simulink model "xblock_half_band_Model"  (Simulink 7.4)
settings: Solver=ode45  StartTime=0.0  StopTime=10.0  RelTol=1e-3
libraries: xbsIndex_r4 x629, casper_library_misc x12
(part 1 of 6)
settings Model: Creator=hong  LastModifiedBy=hong

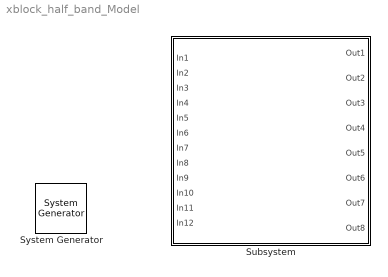
== system xblock_half_band_Model ==
  " System Generator" : xbsIndex_r4/ System Generator  Tag=genX  SystemSampleTime=-1  xilinxfamily=Virtex6  part=xc6vsx315t  speed=-3  package=ff1156  synthesis_tool=XST  clock_wrapper=Clock Enables  directory=./netlist  testbench=off  simulink_period=1  sysclk_period=10  dcm_input_clock_period=10  incr_netlist=off  trim_vbits=Everywhere in SubSystem  dbl_ovrd=According to Block Masks  core_generation=According to Block Masks  run_coregen=off  deprecated_control=off  eval_field=0  block_type=sysgen
      settings: block_version=11.4
  Subsystem : Subsystem

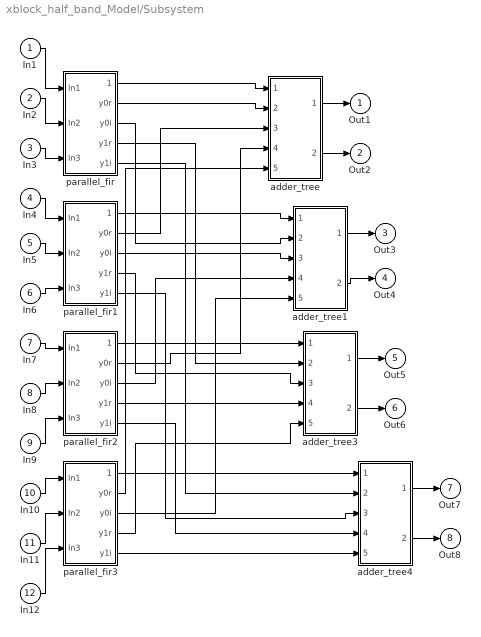
== system xblock_half_band_Model/Subsystem ==
  In1 : Inport
  In2 : Inport  Port=2
  In3 : Inport  Port=3
  In4 : Inport  Port=4
  In5 : Inport  Port=5
  In6 : Inport  Port=6
  In7 : Inport  Port=7
  In8 : Inport  Port=8
  In9 : Inport  Port=9
  In10 : Inport  Port=10
  In11 : Inport  Port=11
  In12 : Inport  Port=12
  adder_tree : Subsystem
  adder_tree1 : Subsystem
  adder_tree3 : Subsystem
  adder_tree4 : Subsystem
  parallel_fir : Subsystem
  parallel_fir1 : Subsystem
  parallel_fir2 : Subsystem
  parallel_fir3 : Subsystem
  Out1 : Outport
  Out2 : Outport  Port=2
  Out3 : Outport  Port=3
  Out4 : Outport  Port=4
  Out5 : Outport  Port=5
  Out6 : Outport  Port=6
  Out7 : Outport  Port=7
  Out8 : Outport  Port=8
  wires:
  parallel_fir3/4(y1r) -> adder_tree3/5(din_4)
  parallel_fir3/2(y0r) -> adder_tree/5(din_4)
  In12/1 -> parallel_fir3/3(In3)
  In10/1 -> parallel_fir3/1(In1)
  parallel_fir2/5(y1i) -> adder_tree4/4(din_3)
  parallel_fir2/3(y0i) -> adder_tree1/4(din_3)
  parallel_fir2/1(sync_out) -> adder_tree3/1(sync)
  In8/1 -> parallel_fir2/2(In2)
  parallel_fir1/4(y1r) -> adder_tree3/3(din_2)
  parallel_fir1/2(y0r) -> adder_tree/3(din_2)
  In6/1 -> parallel_fir1/3(In3)
  In4/1 -> parallel_fir1/1(In1)
  parallel_fir/5(y1i) -> adder_tree4/2(din_1)
  parallel_fir/3(y0i) -> adder_tree1/2(din_1)
  parallel_fir/1(sync_out) -> adder_tree/1(sync)
  In2/1 -> parallel_fir/2(In2)
  adder_tree4/1(sync_out) -> Out7/1
  adder_tree3/2(dout) -> Out6/1
  adder_tree1/1(sync_out) -> Out3/1
  adder_tree/2(dout) -> Out2/1
  adder_tree/1(sync_out) -> Out1/1
  adder_tree1/2(dout) -> Out4/1
  adder_tree3/1(sync_out) -> Out5/1
  adder_tree4/2(dout) -> Out8/1
  In1/1 -> parallel_fir/1(In1)
  In3/1 -> parallel_fir/3(In3)
  parallel_fir/2(y0r) -> adder_tree/2(din_1)
  parallel_fir/4(y1r) -> adder_tree3/2(din_1)
  In5/1 -> parallel_fir1/2(In2)
  parallel_fir1/1(sync_out) -> adder_tree1/1(sync)
  parallel_fir1/3(y0i) -> adder_tree1/3(din_2)
  parallel_fir1/5(y1i) -> adder_tree4/3(din_2)
  In7/1 -> parallel_fir2/1(In1)
  In9/1 -> parallel_fir2/3(In3)
  parallel_fir2/2(y0r) -> adder_tree/4(din_3)
  parallel_fir2/4(y1r) -> adder_tree3/4(din_3)
  In11/1 -> parallel_fir3/2(In2)
  parallel_fir3/1(sync_out) -> adder_tree4/1(sync)
  parallel_fir3/3(y0i) -> adder_tree1/5(din_4)
  parallel_fir3/5(y1i) -> adder_tree4/5(din_4)

== system xblock_half_band_Model/Subsystem/adder_tree ==
  sync : Inport
  din_1 : Inport  Port=2
  din_2 : Inport  Port=3
  din_3 : Inport  Port=4
  din_4 : Inport  Port=5
  adder_0 : xbsIndex_r4/AddSub  mode=Addition  use_carryin=off  use_carryout=off  en=off  latency=1  precision=Full  arith_type=Unsigned  n_bits=16  bin_pt=14  quantization=Truncate  overflow=Saturate  dbl_ovrd=off  use_behavioral_HDL=off  hw_selection=Fabric  pipelined=off  block_type=addsub
  adder_1 : xbsIndex_r4/AddSub  mode=Addition  use_carryin=off  use_carryout=off  en=off  latency=1  precision=Full  arith_type=Unsigned  n_bits=16  bin_pt=14  quantization=Truncate  overflow=Saturate  dbl_ovrd=off  use_behavioral_HDL=off  hw_selection=Fabric  pipelined=off  block_type=addsub
  adder_2 : xbsIndex_r4/AddSub  mode=Addition  use_carryin=off  use_carryout=off  en=off  latency=1  precision=Full  arith_type=Unsigned  n_bits=16  bin_pt=14  quantization=Truncate  overflow=Saturate  dbl_ovrd=off  use_behavioral_HDL=off  hw_selection=Fabric  pipelined=off  block_type=addsub
  sync_delay : xbsIndex_r4/Delay  en=off  latency=2  dbl_ovrd=off  reg_retiming=off  block_type=delay
      settings: block_version=11.4
  zero_in : xbsIndex_r4/Constant  arith_type=Unsigned  const=0  n_bits=18  bin_pt=17  explicit_period=off  period=1  equ=P=C  opselect=C  inp2=PCIN>>17  opr=+  inp1=P  carry=CIN  dbl_ovrd=off  block_type=constant
      settings: block_version=11.4
  sync_out : Outport
  dout : Outport  Port=2
  wires:
  adder_0/1 -> adder_2/2
  din_4/1 -> adder_1/1
  din_1/1 -> adder_0/2
  sync/1 -> sync_delay/1
  sync_delay/1 -> sync_out/1
  din_2/1 -> adder_0/1
  din_3/1 -> adder_1/2
  adder_1/1 -> adder_2/1
  adder_2/1 -> dout/1

== system xblock_half_band_Model/Subsystem/adder_tree1 ==
  sync : Inport
  din_1 : Inport  Port=2
  din_2 : Inport  Port=3
  din_3 : Inport  Port=4
  din_4 : Inport  Port=5
  adder_0 : xbsIndex_r4/AddSub  mode=Addition  use_carryin=off  use_carryout=off  en=off  latency=1  precision=Full  arith_type=Unsigned  n_bits=16  bin_pt=14  quantization=Truncate  overflow=Saturate  dbl_ovrd=off  use_behavioral_HDL=off  hw_selection=Fabric  pipelined=off  block_type=addsub
  adder_1 : xbsIndex_r4/AddSub  mode=Addition  use_carryin=off  use_carryout=off  en=off  latency=1  precision=Full  arith_type=Unsigned  n_bits=16  bin_pt=14  quantization=Truncate  overflow=Saturate  dbl_ovrd=off  use_behavioral_HDL=off  hw_selection=Fabric  pipelined=off  block_type=addsub
  adder_2 : xbsIndex_r4/AddSub  mode=Addition  use_carryin=off  use_carryout=off  en=off  latency=1  precision=Full  arith_type=Unsigned  n_bits=16  bin_pt=14  quantization=Truncate  overflow=Saturate  dbl_ovrd=off  use_behavioral_HDL=off  hw_selection=Fabric  pipelined=off  block_type=addsub
  sync_delay : xbsIndex_r4/Delay  en=off  latency=2  dbl_ovrd=off  reg_retiming=off  block_type=delay
      settings: block_version=11.4
  zero_in : xbsIndex_r4/Constant  arith_type=Unsigned  const=0  n_bits=18  bin_pt=17  explicit_period=off  period=1  equ=P=C  opselect=C  inp2=PCIN>>17  opr=+  inp1=P  carry=CIN  dbl_ovrd=off  block_type=constant
      settings: block_version=11.4
  sync_out : Outport
  dout : Outport  Port=2
  wires:
  adder_0/1 -> adder_2/2
  din_4/1 -> adder_1/1
  din_1/1 -> adder_0/2
  sync/1 -> sync_delay/1
  sync_delay/1 -> sync_out/1
  din_2/1 -> adder_0/1
  din_3/1 -> adder_1/2
  adder_1/1 -> adder_2/1
  adder_2/1 -> dout/1

== system xblock_half_band_Model/Subsystem/adder_tree3 ==
  sync : Inport
  din_1 : Inport  Port=2
  din_2 : Inport  Port=3
  din_3 : Inport  Port=4
  din_4 : Inport  Port=5
  adder_0 : xbsIndex_r4/AddSub  mode=Addition  use_carryin=off  use_carryout=off  en=off  latency=1  precision=Full  arith_type=Unsigned  n_bits=16  bin_pt=14  quantization=Truncate  overflow=Saturate  dbl_ovrd=off  use_behavioral_HDL=off  hw_selection=Fabric  pipelined=off  block_type=addsub
  adder_1 : xbsIndex_r4/AddSub  mode=Addition  use_carryin=off  use_carryout=off  en=off  latency=1  precision=Full  arith_type=Unsigned  n_bits=16  bin_pt=14  quantization=Truncate  overflow=Saturate  dbl_ovrd=off  use_behavioral_HDL=off  hw_selection=Fabric  pipelined=off  block_type=addsub
  adder_2 : xbsIndex_r4/AddSub  mode=Addition  use_carryin=off  use_carryout=off  en=off  latency=1  precision=Full  arith_type=Unsigned  n_bits=16  bin_pt=14  quantization=Truncate  overflow=Saturate  dbl_ovrd=off  use_behavioral_HDL=off  hw_selection=Fabric  pipelined=off  block_type=addsub
  sync_delay : xbsIndex_r4/Delay  en=off  latency=2  dbl_ovrd=off  reg_retiming=off  block_type=delay
      settings: block_version=11.4
  zero_in : xbsIndex_r4/Constant  arith_type=Unsigned  const=0  n_bits=18  bin_pt=17  explicit_period=off  period=1  equ=P=C  opselect=C  inp2=PCIN>>17  opr=+  inp1=P  carry=CIN  dbl_ovrd=off  block_type=constant
      settings: block_version=11.4
  sync_out : Outport
  dout : Outport  Port=2
  wires:
  adder_0/1 -> adder_2/2
  din_4/1 -> adder_1/1
  din_1/1 -> adder_0/2
  sync/1 -> sync_delay/1
  sync_delay/1 -> sync_out/1
  din_2/1 -> adder_0/1
  din_3/1 -> adder_1/2
  adder_1/1 -> adder_2/1
  adder_2/1 -> dout/1

== system xblock_half_band_Model/Subsystem/adder_tree4 ==
  sync : Inport
  din_1 : Inport  Port=2
  din_2 : Inport  Port=3
  din_3 : Inport  Port=4
  din_4 : Inport  Port=5
  adder_0 : xbsIndex_r4/AddSub  mode=Addition  use_carryin=off  use_carryout=off  en=off  latency=1  precision=Full  arith_type=Unsigned  n_bits=16  bin_pt=14  quantization=Truncate  overflow=Saturate  dbl_ovrd=off  use_behavioral_HDL=off  hw_selection=Fabric  pipelined=off  block_type=addsub
  adder_1 : xbsIndex_r4/AddSub  mode=Addition  use_carryin=off  use_carryout=off  en=off  latency=1  precision=Full  arith_type=Unsigned  n_bits=16  bin_pt=14  quantization=Truncate  overflow=Saturate  dbl_ovrd=off  use_behavioral_HDL=off  hw_selection=Fabric  pipelined=off  block_type=addsub
  adder_2 : xbsIndex_r4/AddSub  mode=Addition  use_carryin=off  use_carryout=off  en=off  latency=1  precision=Full  arith_type=Unsigned  n_bits=16  bin_pt=14  quantization=Truncate  overflow=Saturate  dbl_ovrd=off  use_behavioral_HDL=off  hw_selection=Fabric  pipelined=off  block_type=addsub
  sync_delay : xbsIndex_r4/Delay  en=off  latency=2  dbl_ovrd=off  reg_retiming=off  block_type=delay
      settings: block_version=11.4
  zero_in : xbsIndex_r4/Constant  arith_type=Unsigned  const=0  n_bits=18  bin_pt=17  explicit_period=off  period=1  equ=P=C  opselect=C  inp2=PCIN>>17  opr=+  inp1=P  carry=CIN  dbl_ovrd=off  block_type=constant
      settings: block_version=11.4
  sync_out : Outport
  dout : Outport  Port=2
  wires:
  adder_0/1 -> adder_2/2
  din_4/1 -> adder_1/1
  din_1/1 -> adder_0/2
  sync/1 -> sync_delay/1
  sync_delay/1 -> sync_out/1
  din_2/1 -> adder_0/1
  din_3/1 -> adder_1/2
  adder_1/1 -> adder_2/1
  adder_2/1 -> dout/1

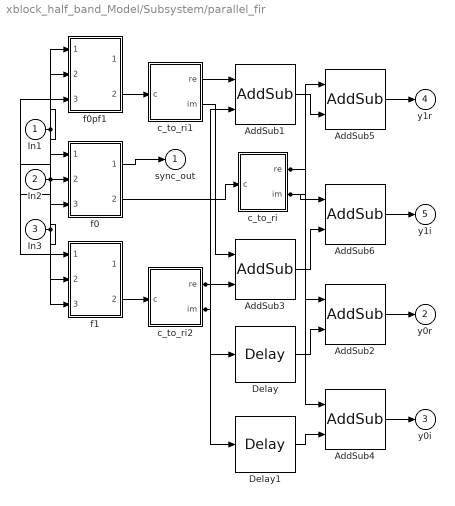
== system xblock_half_band_Model/Subsystem/parallel_fir ==
  In1 : Inport
  In2 : Inport  Port=2
  In3 : Inport  Port=3
  AddSub{1,3,5..6} (4 alike) : xbsIndex_r4/AddSub  mode=Subtraction  use_carryin=off  use_carryout=off  en=off  latency=0  precision=Full  arith_type=Unsigned  n_bits=16  bin_pt=14  quantization=Truncate  overflow=Wrap  dbl_ovrd=off  use_behavioral_HDL=off  hw_selection=Fabric  pipelined=off  block_type=addsub
  AddSub2 : xbsIndex_r4/AddSub  mode=Addition  use_carryin=off  use_carryout=off  en=off  latency=0  precision=Full  arith_type=Unsigned  n_bits=16  bin_pt=14  quantization=Truncate  overflow=Wrap  dbl_ovrd=off  use_behavioral_HDL=off  hw_selection=Fabric  pipelined=off  block_type=addsub
  AddSub4 : xbsIndex_r4/AddSub  mode=Addition  use_carryin=off  use_carryout=off  en=off  latency=0  precision=Full  arith_type=Unsigned  n_bits=16  bin_pt=14  quantization=Truncate  overflow=Wrap  dbl_ovrd=off  use_behavioral_HDL=off  hw_selection=Fabric  pipelined=off  block_type=addsub
  Delay : xbsIndex_r4/Delay  en=off  latency=1  dbl_ovrd=off  reg_retiming=off  block_type=delay
      settings: block_version=11.4
  Delay1 : xbsIndex_r4/Delay  en=off  latency=1  dbl_ovrd=off  reg_retiming=off  block_type=delay
      settings: block_version=11.4
  c_to_ri : Subsystem
  c_to_ri1 : Subsystem
  c_to_ri2 : Subsystem
  f0 : Subsystem
  f0pf1 : Subsystem
  f1 : Subsystem
  sync_out : Outport
  y0r : Outport  Port=2
  y0i : Outport  Port=3
  y1r : Outport  Port=4
  y1i : Outport  Port=5
  wires:
  c_to_ri/1(re) -> AddSub5/1, AddSub2/1
  c_to_ri/2(im) -> AddSub4/1, AddSub6/1
  c_to_ri2/1(re) -> Delay/1, AddSub1/2
  c_to_ri2/2(im) -> AddSub3/2, Delay1/1
  In1/1 -> f1/1(sync_in), f0/1(sync_in), f0pf1/1(sync_in)
  In2/1 -> f0pf1/2(real1), f0/2(real1), f1/2(real1)
  In3/1 -> f1/3(imag1), f0/3(imag1), f0pf1/3(imag1)
  f0pf1/2(dout) -> c_to_ri1/1(c)
  f0/1(sync_out) -> sync_out/1
  c_to_ri1/2(im) -> AddSub3/1
  Delay1/1 -> AddSub4/2
  Delay/1 -> AddSub2/2
  AddSub6/1 -> y1i/1
  AddSub1/1 -> AddSub5/2
  AddSub4/1 -> y0i/1
  AddSub2/1 -> y0r/1
  AddSub5/1 -> y1r/1
  AddSub3/1 -> AddSub6/2
  c_to_ri1/1(re) -> AddSub1/1
  f0/2(dout) -> c_to_ri/1(c)
  f1/2(dout) -> c_to_ri2/1(c)

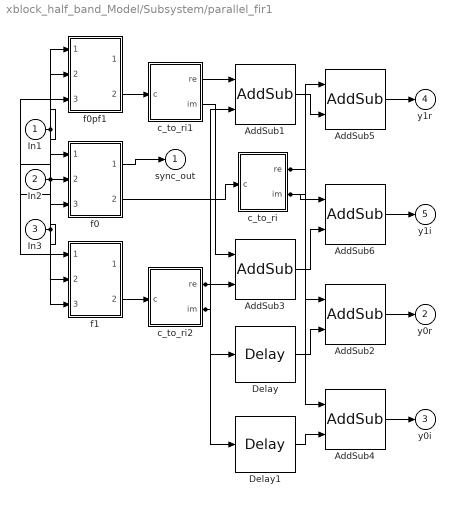
== system xblock_half_band_Model/Subsystem/parallel_fir1 ==
  In1 : Inport
  In2 : Inport  Port=2
  In3 : Inport  Port=3
  AddSub{1,3,5..6} (4 alike) : xbsIndex_r4/AddSub  mode=Subtraction  use_carryin=off  use_carryout=off  en=off  latency=0  precision=Full  arith_type=Unsigned  n_bits=16  bin_pt=14  quantization=Truncate  overflow=Wrap  dbl_ovrd=off  use_behavioral_HDL=off  hw_selection=Fabric  pipelined=off  block_type=addsub
  AddSub2 : xbsIndex_r4/AddSub  mode=Addition  use_carryin=off  use_carryout=off  en=off  latency=0  precision=Full  arith_type=Unsigned  n_bits=16  bin_pt=14  quantization=Truncate  overflow=Wrap  dbl_ovrd=off  use_behavioral_HDL=off  hw_selection=Fabric  pipelined=off  block_type=addsub
  AddSub4 : xbsIndex_r4/AddSub  mode=Addition  use_carryin=off  use_carryout=off  en=off  latency=0  precision=Full  arith_type=Unsigned  n_bits=16  bin_pt=14  quantization=Truncate  overflow=Wrap  dbl_ovrd=off  use_behavioral_HDL=off  hw_selection=Fabric  pipelined=off  block_type=addsub
  Delay : xbsIndex_r4/Delay  en=off  latency=1  dbl_ovrd=off  reg_retiming=off  block_type=delay
      settings: block_version=11.4
  Delay1 : xbsIndex_r4/Delay  en=off  latency=1  dbl_ovrd=off  reg_retiming=off  block_type=delay
      settings: block_version=11.4
  c_to_ri : Subsystem
  c_to_ri1 : Subsystem
  c_to_ri2 : Subsystem
  f0 : Subsystem
  f0pf1 : Subsystem
  f1 : Subsystem
  sync_out : Outport
  y0r : Outport  Port=2
  y0i : Outport  Port=3
  y1r : Outport  Port=4
  y1i : Outport  Port=5
  wires:
  c_to_ri/1(re) -> AddSub5/1, AddSub2/1
  c_to_ri/2(im) -> AddSub4/1, AddSub6/1
  c_to_ri2/1(re) -> Delay/1, AddSub1/2
  c_to_ri2/2(im) -> AddSub3/2, Delay1/1
  In1/1 -> f1/1(sync_in), f0/1(sync_in), f0pf1/1(sync_in)
  In2/1 -> f0pf1/2(real1), f0/2(real1), f1/2(real1)
  In3/1 -> f1/3(imag1), f0/3(imag1), f0pf1/3(imag1)
  f0pf1/2(dout) -> c_to_ri1/1(c)
  f0/1(sync_out) -> sync_out/1
  c_to_ri1/2(im) -> AddSub3/1
  Delay1/1 -> AddSub4/2
  Delay/1 -> AddSub2/2
  AddSub6/1 -> y1i/1
  AddSub1/1 -> AddSub5/2
  AddSub4/1 -> y0i/1
  AddSub2/1 -> y0r/1
  AddSub5/1 -> y1r/1
  AddSub3/1 -> AddSub6/2
  c_to_ri1/1(re) -> AddSub1/1
  f0/2(dout) -> c_to_ri/1(c)
  f1/2(dout) -> c_to_ri2/1(c)

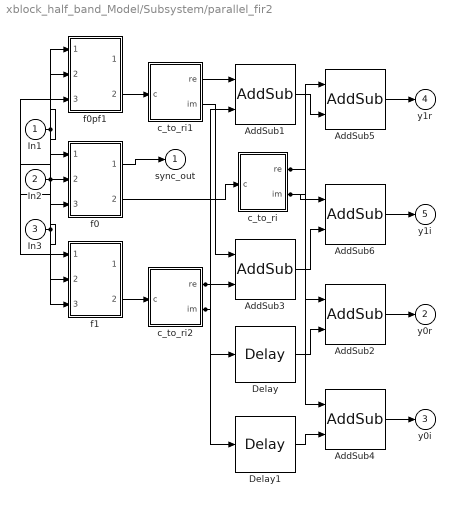
== system xblock_half_band_Model/Subsystem/parallel_fir2 ==
  In1 : Inport
  In2 : Inport  Port=2
  In3 : Inport  Port=3
  AddSub{1,3,5..6} (4 alike) : xbsIndex_r4/AddSub  mode=Subtraction  use_carryin=off  use_carryout=off  en=off  latency=0  precision=Full  arith_type=Unsigned  n_bits=16  bin_pt=14  quantization=Truncate  overflow=Wrap  dbl_ovrd=off  use_behavioral_HDL=off  hw_selection=Fabric  pipelined=off  block_type=addsub
  AddSub2 : xbsIndex_r4/AddSub  mode=Addition  use_carryin=off  use_carryout=off  en=off  latency=0  precision=Full  arith_type=Unsigned  n_bits=16  bin_pt=14  quantization=Truncate  overflow=Wrap  dbl_ovrd=off  use_behavioral_HDL=off  hw_selection=Fabric  pipelined=off  block_type=addsub
  AddSub4 : xbsIndex_r4/AddSub  mode=Addition  use_carryin=off  use_carryout=off  en=off  latency=0  precision=Full  arith_type=Unsigned  n_bits=16  bin_pt=14  quantization=Truncate  overflow=Wrap  dbl_ovrd=off  use_behavioral_HDL=off  hw_selection=Fabric  pipelined=off  block_type=addsub
  Delay : xbsIndex_r4/Delay  en=off  latency=1  dbl_ovrd=off  reg_retiming=off  block_type=delay
      settings: block_version=11.4
  Delay1 : xbsIndex_r4/Delay  en=off  latency=1  dbl_ovrd=off  reg_retiming=off  block_type=delay
      settings: block_version=11.4
  c_to_ri : Subsystem
  c_to_ri1 : Subsystem
  c_to_ri2 : Subsystem
  f0 : Subsystem
  f0pf1 : Subsystem
  f1 : Subsystem
  sync_out : Outport
  y0r : Outport  Port=2
  y0i : Outport  Port=3
  y1r : Outport  Port=4
  y1i : Outport  Port=5
  wires:
  c_to_ri/1(re) -> AddSub5/1, AddSub2/1
  c_to_ri/2(im) -> AddSub4/1, AddSub6/1
  c_to_ri2/1(re) -> Delay/1, AddSub1/2
  c_to_ri2/2(im) -> AddSub3/2, Delay1/1
  In1/1 -> f1/1(sync_in), f0/1(sync_in), f0pf1/1(sync_in)
  In2/1 -> f0pf1/2(real1), f0/2(real1), f1/2(real1)
  In3/1 -> f1/3(imag1), f0/3(imag1), f0pf1/3(imag1)
  f0pf1/2(dout) -> c_to_ri1/1(c)
  f0/1(sync_out) -> sync_out/1
  c_to_ri1/2(im) -> AddSub3/1
  Delay1/1 -> AddSub4/2
  Delay/1 -> AddSub2/2
  AddSub6/1 -> y1i/1
  AddSub1/1 -> AddSub5/2
  AddSub4/1 -> y0i/1
  AddSub2/1 -> y0r/1
  AddSub5/1 -> y1r/1
  AddSub3/1 -> AddSub6/2
  c_to_ri1/1(re) -> AddSub1/1
  f0/2(dout) -> c_to_ri/1(c)
  f1/2(dout) -> c_to_ri2/1(c)

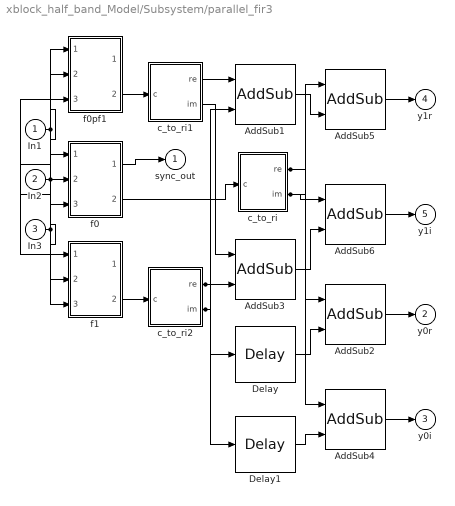
== system xblock_half_band_Model/Subsystem/parallel_fir3 ==
  In1 : Inport
  In2 : Inport  Port=2
  In3 : Inport  Port=3
  AddSub{1,3,5..6} (4 alike) : xbsIndex_r4/AddSub  mode=Subtraction  use_carryin=off  use_carryout=off  en=off  latency=0  precision=Full  arith_type=Unsigned  n_bits=16  bin_pt=14  quantization=Truncate  overflow=Wrap  dbl_ovrd=off  use_behavioral_HDL=off  hw_selection=Fabric  pipelined=off  block_type=addsub
  AddSub2 : xbsIndex_r4/AddSub  mode=Addition  use_carryin=off  use_carryout=off  en=off  latency=0  precision=Full  arith_type=Unsigned  n_bits=16  bin_pt=14  quantization=Truncate  overflow=Wrap  dbl_ovrd=off  use_behavioral_HDL=off  hw_selection=Fabric  pipelined=off  block_type=addsub
  AddSub4 : xbsIndex_r4/AddSub  mode=Addition  use_carryin=off  use_carryout=off  en=off  latency=0  precision=Full  arith_type=Unsigned  n_bits=16  bin_pt=14  quantization=Truncate  overflow=Wrap  dbl_ovrd=off  use_behavioral_HDL=off  hw_selection=Fabric  pipelined=off  block_type=addsub
  Delay : xbsIndex_r4/Delay  en=off  latency=1  dbl_ovrd=off  reg_retiming=off  block_type=delay
      settings: block_version=11.4
  Delay1 : xbsIndex_r4/Delay  en=off  latency=1  dbl_ovrd=off  reg_retiming=off  block_type=delay
      settings: block_version=11.4
  c_to_ri : Subsystem
  c_to_ri1 : Subsystem
  c_to_ri2 : Subsystem
  f0 : Subsystem
  f0pf1 : Subsystem
  f1 : Subsystem
  sync_out : Outport
  y0r : Outport  Port=2
  y0i : Outport  Port=3
  y1r : Outport  Port=4
  y1i : Outport  Port=5
  wires:
  c_to_ri/1(re) -> AddSub5/1, AddSub2/1
  c_to_ri/2(im) -> AddSub4/1, AddSub6/1
  c_to_ri2/1(re) -> Delay/1, AddSub1/2
  c_to_ri2/2(im) -> AddSub3/2, Delay1/1
  In1/1 -> f1/1(sync_in), f0/1(sync_in), f0pf1/1(sync_in)
  In2/1 -> f0pf1/2(real1), f0/2(real1), f1/2(real1)
  In3/1 -> f1/3(imag1), f0/3(imag1), f0pf1/3(imag1)
  f0pf1/2(dout) -> c_to_ri1/1(c)
  f0/1(sync_out) -> sync_out/1
  c_to_ri1/2(im) -> AddSub3/1
  Delay1/1 -> AddSub4/2
  Delay/1 -> AddSub2/2
  AddSub6/1 -> y1i/1
  AddSub1/1 -> AddSub5/2
  AddSub4/1 -> y0i/1
  AddSub2/1 -> y0r/1
  AddSub5/1 -> y1r/1
  AddSub3/1 -> AddSub6/2
  c_to_ri1/1(re) -> AddSub1/1
  f0/2(dout) -> c_to_ri/1(c)
  f1/2(dout) -> c_to_ri2/1(c)

== system xblock_half_band_Model/Subsystem/parallel_fir/c_to_ri ==
  c : Inport
  force_im : xbsIndex_r4/Reinterpret  force_arith_type=on  arith_type="Signed  (2's comp)"  force_bin_pt=on  bin_pt=7  block_type=reinterpret
      settings: infoedit="Changes signal type without altering the binary representation.   You can changed the signal between signed and unsigned, and relocate the binary point.<br><br>Hardware notes: In hardware this block costs nothing.<br><br>Example:  Suppose the input is 6 bits wide, signed, with 2 fractional bits, and the output is forced to unsigned with 0 fractional bits.  Then an input of -2.0 (1110.00 in binary 2's complement) becomes an output of 56 (111000 in binary)."
  force_re : xbsIndex_r4/Reinterpret  force_arith_type=on  arith_type="Signed  (2's comp)"  force_bin_pt=on  bin_pt=7  block_type=reinterpret
      settings: infoedit="Changes signal type without altering the binary representation.   You can changed the signal between signed and unsigned, and relocate the binary point.<br><br>Hardware notes: In hardware this block costs nothing.<br><br>Example:  Suppose the input is 6 bits wide, signed, with 2 fractional bits, and the output is forced to unsigned with 0 fractional bits.  Then an input of -2.0 (1110.00 in binary 2's complement) becomes an output of 56 (111000 in binary)."
  slice_im : xbsIndex_r4/Slice  nbits=8  boolean_output=off  mode=Lower Bit Location + Width  bit1=0  base1=MSB of Input  bit0=0  base0=LSB of Input  dbl_ovrd=off  block_type=slice
  slice_re : xbsIndex_r4/Slice  nbits=8  boolean_output=off  mode=Upper Bit Location + Width  bit1=0  base1=MSB of Input  bit0=0  base0=LSB of Input  dbl_ovrd=off  block_type=slice
  re : Outport
  im : Outport  Port=2
  wires:
  c/1 -> slice_re/1, slice_im/1
  slice_im/1 -> force_im/1
  force_im/1 -> im/1
  force_re/1 -> re/1
  slice_re/1 -> force_re/1

== system xblock_half_band_Model/Subsystem/parallel_fir/c_to_ri1 ==
  c : Inport
  force_im : xbsIndex_r4/Reinterpret  force_arith_type=on  arith_type="Signed  (2's comp)"  force_bin_pt=on  bin_pt=7  block_type=reinterpret
      settings: infoedit="Changes signal type without altering the binary representation.   You can changed the signal between signed and unsigned, and relocate the binary point.<br><br>Hardware notes: In hardware this block costs nothing.<br><br>Example:  Suppose the input is 6 bits wide, signed, with 2 fractional bits, and the output is forced to unsigned with 0 fractional bits.  Then an input of -2.0 (1110.00 in binary 2's complement) becomes an output of 56 (111000 in binary)."
  force_re : xbsIndex_r4/Reinterpret  force_arith_type=on  arith_type="Signed  (2's comp)"  force_bin_pt=on  bin_pt=7  block_type=reinterpret
      settings: infoedit="Changes signal type without altering the binary representation.   You can changed the signal between signed and unsigned, and relocate the binary point.<br><br>Hardware notes: In hardware this block costs nothing.<br><br>Example:  Suppose the input is 6 bits wide, signed, with 2 fractional bits, and the output is forced to unsigned with 0 fractional bits.  Then an input of -2.0 (1110.00 in binary 2's complement) becomes an output of 56 (111000 in binary)."
  slice_im : xbsIndex_r4/Slice  nbits=8  boolean_output=off  mode=Lower Bit Location + Width  bit1=0  base1=MSB of Input  bit0=0  base0=LSB of Input  dbl_ovrd=off  block_type=slice
  slice_re : xbsIndex_r4/Slice  nbits=8  boolean_output=off  mode=Upper Bit Location + Width  bit1=0  base1=MSB of Input  bit0=0  base0=LSB of Input  dbl_ovrd=off  block_type=slice
  re : Outport
  im : Outport  Port=2
  wires:
  c/1 -> slice_re/1, slice_im/1
  slice_im/1 -> force_im/1
  force_im/1 -> im/1
  force_re/1 -> re/1
  slice_re/1 -> force_re/1

== system xblock_half_band_Model/Subsystem/parallel_fir/c_to_ri2 ==
  c : Inport
  force_im : xbsIndex_r4/Reinterpret  force_arith_type=on  arith_type="Signed  (2's comp)"  force_bin_pt=on  bin_pt=7  block_type=reinterpret
      settings: infoedit="Changes signal type without altering the binary representation.   You can changed the signal between signed and unsigned, and relocate the binary point.<br><br>Hardware notes: In hardware this block costs nothing.<br><br>Example:  Suppose the input is 6 bits wide, signed, with 2 fractional bits, and the output is forced to unsigned with 0 fractional bits.  Then an input of -2.0 (1110.00 in binary 2's complement) becomes an output of 56 (111000 in binary)."
  force_re : xbsIndex_r4/Reinterpret  force_arith_type=on  arith_type="Signed  (2's comp)"  force_bin_pt=on  bin_pt=7  block_type=reinterpret
      settings: infoedit="Changes signal type without altering the binary representation.   You can changed the signal between signed and unsigned, and relocate the binary point.<br><br>Hardware notes: In hardware this block costs nothing.<br><br>Example:  Suppose the input is 6 bits wide, signed, with 2 fractional bits, and the output is forced to unsigned with 0 fractional bits.  Then an input of -2.0 (1110.00 in binary 2's complement) becomes an output of 56 (111000 in binary)."
  slice_im : xbsIndex_r4/Slice  nbits=8  boolean_output=off  mode=Lower Bit Location + Width  bit1=0  base1=MSB of Input  bit0=0  base0=LSB of Input  dbl_ovrd=off  block_type=slice
  slice_re : xbsIndex_r4/Slice  nbits=8  boolean_output=off  mode=Upper Bit Location + Width  bit1=0  base1=MSB of Input  bit0=0  base0=LSB of Input  dbl_ovrd=off  block_type=slice
  re : Outport
  im : Outport  Port=2
  wires:
  c/1 -> slice_re/1, slice_im/1
  slice_im/1 -> force_im/1
  force_im/1 -> im/1
  force_re/1 -> re/1
  slice_re/1 -> force_re/1

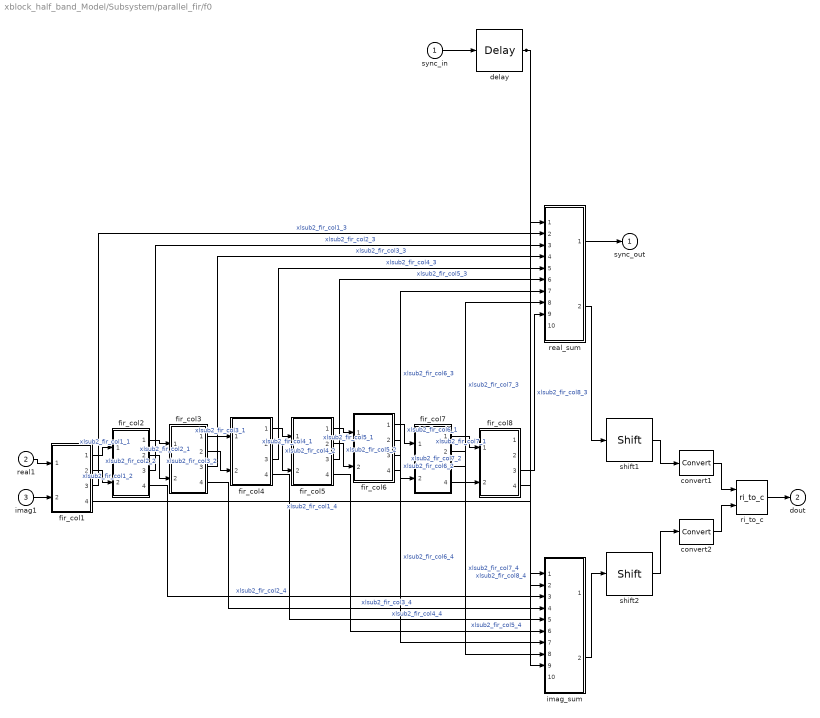
== system xblock_half_band_Model/Subsystem/parallel_fir/f0 ==
  sync_in : Inport
  real1 : Inport  Port=2
  imag1 : Inport  Port=3
  convert1 : xbsIndex_r4/Convert  arith_type="Signed  (2's comp)"  n_bits=4  bin_pt=3  quantization=Truncate  overflow=Wrap  latency=1  dbl_ovrd=off  pipeline=off  block_type=convert
      settings: block_version=11.4
  convert2 : xbsIndex_r4/Convert  arith_type="Signed  (2's comp)"  n_bits=4  bin_pt=3  quantization=Truncate  overflow=Wrap  latency=1  dbl_ovrd=off  pipeline=off  block_type=convert
      settings: block_version=11.4
  delay : xbsIndex_r4/Delay  en=off  latency=3  dbl_ovrd=off  reg_retiming=off  block_type=delay
      settings: block_version=11.4
  fir_col1 : Subsystem
  fir_col2 : Subsystem
  fir_col3 : Subsystem
  fir_col4 : Subsystem
  fir_col5 : Subsystem
  fir_col6 : Subsystem
  fir_col7 : Subsystem
  fir_col8 : Subsystem
  imag_sum : Subsystem
  real_sum : Subsystem
  ri_to_c : casper_library_misc/ri_to_c  SystemSampleTime=-1
  shift1 : xbsIndex_r4/Shift  shift_dir=Left  shift_bits=1  en=off  latency=0  precision=Full  arith_type="Signed  (2's comp)"  n_bits=16  bin_pt=14  quantization=Truncate  overflow=Wrap  dbl_ovrd=off  block_type=shift
  shift2 : xbsIndex_r4/Shift  shift_dir=Left  shift_bits=1  en=off  latency=0  precision=Full  arith_type="Signed  (2's comp)"  n_bits=16  bin_pt=14  quantization=Truncate  overflow=Wrap  dbl_ovrd=off  block_type=shift
  sync_out : Outport
  dout : Outport  Port=2
  wires:
  delay/1 -> real_sum/1(sync), imag_sum/1(sync)
  imag_sum/2(dout) -> shift2/1
  shift1/1 -> convert1/1
  convert2/1 -> ri_to_c/2
  fir_col8/3(real_sum) -> real_sum/9(din_8)  "xlsub2_fir_col8_3"
  fir_col6/3(real_sum) -> real_sum/7(din_6)  "xlsub2_fir_col6_3"
  fir_col4/3(real_sum) -> real_sum/5(din_4)  "xlsub2_fir_col4_3"
  fir_col2/3(real_sum) -> real_sum/3(din_2)  "xlsub2_fir_col2_3"
  fir_col8/4(imag_sum) -> imag_sum/9(din_8)  "xlsub2_fir_col8_4"
  fir_col6/4(imag_sum) -> imag_sum/7(din_6)  "xlsub2_fir_col6_4"
  fir_col4/4(imag_sum) -> imag_sum/5(din_4)  "xlsub2_fir_col4_4"
  fir_col2/4(imag_sum) -> imag_sum/3(din_2)  "xlsub2_fir_col2_4"
  fir_col7/2(imag_out1) -> fir_col8/2(imag1)  "xlsub2_fir_col7_2"
  fir_col6/1(real_out1) -> fir_col7/1(real1)  "xlsub2_fir_col6_1"
  fir_col5/2(imag_out1) -> fir_col6/2(imag1)  "xlsub2_fir_col5_2"
  fir_col4/1(real_out1) -> fir_col5/1(real1)  "xlsub2_fir_col4_1"
  fir_col3/2(imag_out1) -> fir_col4/2(imag1)  "xlsub2_fir_col3_2"
  fir_col2/1(real_out1) -> fir_col3/1(real1)  "xlsub2_fir_col2_1"
  fir_col1/2(imag_out1) -> fir_col2/2(imag1)  "xlsub2_fir_col1_2"
  real1/1 -> fir_col1/1(real1)
  sync_in/1 -> delay/1
  imag1/1 -> fir_col1/2(imag1)
  fir_col1/1(real_out1) -> fir_col2/1(real1)  "xlsub2_fir_col1_1"
  fir_col2/2(imag_out1) -> fir_col3/2(imag1)  "xlsub2_fir_col2_2"
  fir_col3/1(real_out1) -> fir_col4/1(real1)  "xlsub2_fir_col3_1"
  fir_col4/2(imag_out1) -> fir_col5/2(imag1)  "xlsub2_fir_col4_2"
  fir_col5/1(real_out1) -> fir_col6/1(real1)  "xlsub2_fir_col5_1"
  fir_col6/2(imag_out1) -> fir_col7/2(imag1)  "xlsub2_fir_col6_2"
  fir_col7/1(real_out1) -> fir_col8/1(real1)  "xlsub2_fir_col7_1"
  fir_col1/4(imag_sum) -> imag_sum/2(din_1)  "xlsub2_fir_col1_4"
  fir_col3/4(imag_sum) -> imag_sum/4(din_3)  "xlsub2_fir_col3_4"
  fir_col5/4(imag_sum) -> imag_sum/6(din_5)  "xlsub2_fir_col5_4"
  fir_col7/4(imag_sum) -> imag_sum/8(din_7)  "xlsub2_fir_col7_4"
  fir_col1/3(real_sum) -> real_sum/2(din_1)  "xlsub2_fir_col1_3"
  fir_col3/3(real_sum) -> real_sum/4(din_3)  "xlsub2_fir_col3_3"
  fir_col5/3(real_sum) -> real_sum/6(din_5)  "xlsub2_fir_col5_3"
  fir_col7/3(real_sum) -> real_sum/8(din_7)  "xlsub2_fir_col7_3"
  real_sum/1(sync_out) -> sync_out/1
  convert1/1 -> ri_to_c/1
  ri_to_c/1 -> dout/1
  real_sum/2(dout) -> shift1/1
  shift2/1 -> convert2/1

== system xblock_half_band_Model/Subsystem/parallel_fir/f0pf1 ==
  sync_in : Inport
  real1 : Inport  Port=2
  imag1 : Inport  Port=3
  convert1 : xbsIndex_r4/Convert  arith_type="Signed  (2's comp)"  n_bits=4  bin_pt=3  quantization=Truncate  overflow=Wrap  latency=1  dbl_ovrd=off  pipeline=off  block_type=convert
      settings: block_version=11.4
  convert2 : xbsIndex_r4/Convert  arith_type="Signed  (2's comp)"  n_bits=4  bin_pt=3  quantization=Truncate  overflow=Wrap  latency=1  dbl_ovrd=off  pipeline=off  block_type=convert
      settings: block_version=11.4
  delay : xbsIndex_r4/Delay  en=off  latency=3  dbl_ovrd=off  reg_retiming=off  block_type=delay
      settings: block_version=11.4
  fir_col1 : Subsystem
  fir_col2 : Subsystem
  fir_col3 : Subsystem
  fir_col4 : Subsystem
  fir_col5 : Subsystem
  imag_sum : Subsystem
  real_sum : Subsystem
  ri_to_c : casper_library_misc/ri_to_c  SystemSampleTime=-1
  shift1 : xbsIndex_r4/Shift  shift_dir=Left  shift_bits=1  en=off  latency=0  precision=Full  arith_type="Signed  (2's comp)"  n_bits=16  bin_pt=14  quantization=Truncate  overflow=Wrap  dbl_ovrd=off  block_type=shift
  shift2 : xbsIndex_r4/Shift  shift_dir=Left  shift_bits=1  en=off  latency=0  precision=Full  arith_type="Signed  (2's comp)"  n_bits=16  bin_pt=14  quantization=Truncate  overflow=Wrap  dbl_ovrd=off  block_type=shift
  sync_out : Outport
  dout : Outport  Port=2
  wires:
  delay/1 -> imag_sum/1(sync), real_sum/1(sync)
  imag_sum/2(dout) -> shift2/1
  shift1/1 -> convert1/1
  convert2/1 -> ri_to_c/2
  fir_col5/3(real_sum) -> real_sum/6(din_5)  "xlsub2_fir_col5_3"
  fir_col3/3(real_sum) -> real_sum/4(din_3)  "xlsub2_fir_col3_3"
  fir_col1/3(real_sum) -> real_sum/2(din_1)  "xlsub2_fir_col1_3"
  fir_col4/4(imag_sum) -> imag_sum/5(din_4)  "xlsub2_fir_col4_4"
  fir_col2/4(imag_sum) -> imag_sum/3(din_2)  "xlsub2_fir_col2_4"
  fir_col4/2(imag_out1) -> fir_col5/2(imag1)  "xlsub2_fir_col4_2"
  fir_col3/1(real_out1) -> fir_col4/1(real1)  "xlsub2_fir_col3_1"
  fir_col2/2(imag_out1) -> fir_col3/2(imag1)  "xlsub2_fir_col2_2"
  fir_col1/1(real_out1) -> fir_col2/1(real1)  "xlsub2_fir_col1_1"
  imag1/1 -> fir_col1/2(imag1)
  sync_in/1 -> delay/1
  real1/1 -> fir_col1/1(real1)
  fir_col1/2(imag_out1) -> fir_col2/2(imag1)  "xlsub2_fir_col1_2"
  fir_col2/1(real_out1) -> fir_col3/1(real1)  "xlsub2_fir_col2_1"
  fir_col3/2(imag_out1) -> fir_col4/2(imag1)  "xlsub2_fir_col3_2"
  fir_col4/1(real_out1) -> fir_col5/1(real1)  "xlsub2_fir_col4_1"
  fir_col1/4(imag_sum) -> imag_sum/2(din_1)  "xlsub2_fir_col1_4"
  fir_col3/4(imag_sum) -> imag_sum/4(din_3)  "xlsub2_fir_col3_4"
  fir_col5/4(imag_sum) -> imag_sum/6(din_5)  "xlsub2_fir_col5_4"
  fir_col2/3(real_sum) -> real_sum/3(din_2)  "xlsub2_fir_col2_3"
  fir_col4/3(real_sum) -> real_sum/5(din_4)  "xlsub2_fir_col4_3"
  real_sum/1(sync_out) -> sync_out/1
  convert1/1 -> ri_to_c/1
  ri_to_c/1 -> dout/1
  real_sum/2(dout) -> shift1/1
  shift2/1 -> convert2/1

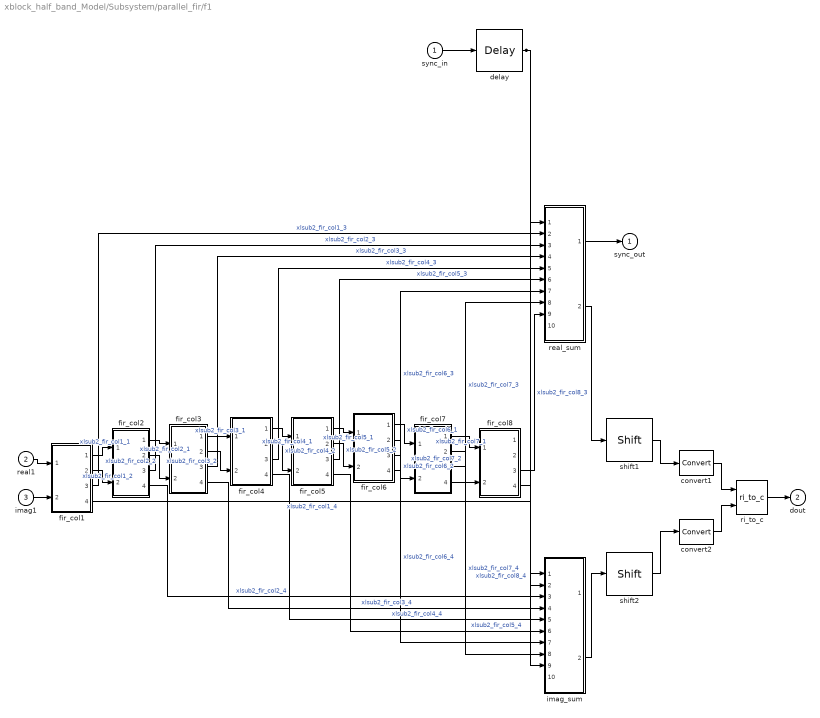
== system xblock_half_band_Model/Subsystem/parallel_fir/f1 ==
  sync_in : Inport
  real1 : Inport  Port=2
  imag1 : Inport  Port=3
  convert1 : xbsIndex_r4/Convert  arith_type="Signed  (2's comp)"  n_bits=4  bin_pt=3  quantization=Truncate  overflow=Wrap  latency=1  dbl_ovrd=off  pipeline=off  block_type=convert
      settings: block_version=11.4
  convert2 : xbsIndex_r4/Convert  arith_type="Signed  (2's comp)"  n_bits=4  bin_pt=3  quantization=Truncate  overflow=Wrap  latency=1  dbl_ovrd=off  pipeline=off  block_type=convert
      settings: block_version=11.4
  delay : xbsIndex_r4/Delay  en=off  latency=3  dbl_ovrd=off  reg_retiming=off  block_type=delay
      settings: block_version=11.4
  fir_col1 : Subsystem
  fir_col2 : Subsystem
  fir_col3 : Subsystem
  fir_col4 : Subsystem
  fir_col5 : Subsystem
  fir_col6 : Subsystem
  fir_col7 : Subsystem
  fir_col8 : Subsystem
  imag_sum : Subsystem
  real_sum : Subsystem
  ri_to_c : casper_library_misc/ri_to_c  SystemSampleTime=-1
  shift1 : xbsIndex_r4/Shift  shift_dir=Left  shift_bits=1  en=off  latency=0  precision=Full  arith_type="Signed  (2's comp)"  n_bits=16  bin_pt=14  quantization=Truncate  overflow=Wrap  dbl_ovrd=off  block_type=shift
  shift2 : xbsIndex_r4/Shift  shift_dir=Left  shift_bits=1  en=off  latency=0  precision=Full  arith_type="Signed  (2's comp)"  n_bits=16  bin_pt=14  quantization=Truncate  overflow=Wrap  dbl_ovrd=off  block_type=shift
  sync_out : Outport
  dout : Outport  Port=2
  wires:
  delay/1 -> real_sum/1(sync), imag_sum/1(sync)
  imag_sum/2(dout) -> shift2/1
  shift1/1 -> convert1/1
  convert2/1 -> ri_to_c/2
  fir_col8/3(real_sum) -> real_sum/9(din_8)  "xlsub2_fir_col8_3"
  fir_col6/3(real_sum) -> real_sum/7(din_6)  "xlsub2_fir_col6_3"
  fir_col4/3(real_sum) -> real_sum/5(din_4)  "xlsub2_fir_col4_3"
  fir_col2/3(real_sum) -> real_sum/3(din_2)  "xlsub2_fir_col2_3"
  fir_col8/4(imag_sum) -> imag_sum/9(din_8)  "xlsub2_fir_col8_4"
  fir_col6/4(imag_sum) -> imag_sum/7(din_6)  "xlsub2_fir_col6_4"
  fir_col4/4(imag_sum) -> imag_sum/5(din_4)  "xlsub2_fir_col4_4"
  fir_col2/4(imag_sum) -> imag_sum/3(din_2)  "xlsub2_fir_col2_4"
  fir_col7/2(imag_out1) -> fir_col8/2(imag1)  "xlsub2_fir_col7_2"
  fir_col6/1(real_out1) -> fir_col7/1(real1)  "xlsub2_fir_col6_1"
  fir_col5/2(imag_out1) -> fir_col6/2(imag1)  "xlsub2_fir_col5_2"
  fir_col4/1(real_out1) -> fir_col5/1(real1)  "xlsub2_fir_col4_1"
  fir_col3/2(imag_out1) -> fir_col4/2(imag1)  "xlsub2_fir_col3_2"
  fir_col2/1(real_out1) -> fir_col3/1(real1)  "xlsub2_fir_col2_1"
  fir_col1/2(imag_out1) -> fir_col2/2(imag1)  "xlsub2_fir_col1_2"
  real1/1 -> fir_col1/1(real1)
  sync_in/1 -> delay/1
  imag1/1 -> fir_col1/2(imag1)
  fir_col1/1(real_out1) -> fir_col2/1(real1)  "xlsub2_fir_col1_1"
  fir_col2/2(imag_out1) -> fir_col3/2(imag1)  "xlsub2_fir_col2_2"
  fir_col3/1(real_out1) -> fir_col4/1(real1)  "xlsub2_fir_col3_1"
  fir_col4/2(imag_out1) -> fir_col5/2(imag1)  "xlsub2_fir_col4_2"
  fir_col5/1(real_out1) -> fir_col6/1(real1)  "xlsub2_fir_col5_1"
  fir_col6/2(imag_out1) -> fir_col7/2(imag1)  "xlsub2_fir_col6_2"
  fir_col7/1(real_out1) -> fir_col8/1(real1)  "xlsub2_fir_col7_1"
  fir_col1/4(imag_sum) -> imag_sum/2(din_1)  "xlsub2_fir_col1_4"
  fir_col3/4(imag_sum) -> imag_sum/4(din_3)  "xlsub2_fir_col3_4"
  fir_col5/4(imag_sum) -> imag_sum/6(din_5)  "xlsub2_fir_col5_4"
  fir_col7/4(imag_sum) -> imag_sum/8(din_7)  "xlsub2_fir_col7_4"
  fir_col1/3(real_sum) -> real_sum/2(din_1)  "xlsub2_fir_col1_3"
  fir_col3/3(real_sum) -> real_sum/4(din_3)  "xlsub2_fir_col3_3"
  fir_col5/3(real_sum) -> real_sum/6(din_5)  "xlsub2_fir_col5_3"
  fir_col7/3(real_sum) -> real_sum/8(din_7)  "xlsub2_fir_col7_3"
  real_sum/1(sync_out) -> sync_out/1
  convert1/1 -> ri_to_c/1
  ri_to_c/1 -> dout/1
  real_sum/2(dout) -> shift1/1
  shift2/1 -> convert2/1

== system xblock_half_band_Model/Subsystem/parallel_fir1/c_to_ri ==
  c : Inport
  force_im : xbsIndex_r4/Reinterpret  force_arith_type=on  arith_type="Signed  (2's comp)"  force_bin_pt=on  bin_pt=7  block_type=reinterpret
      settings: infoedit="Changes signal type without altering the binary representation.   You can changed the signal between signed and unsigned, and relocate the binary point.<br><br>Hardware notes: In hardware this block costs nothing.<br><br>Example:  Suppose the input is 6 bits wide, signed, with 2 fractional bits, and the output is forced to unsigned with 0 fractional bits.  Then an input of -2.0 (1110.00 in binary 2's complement) becomes an output of 56 (111000 in binary)."
  force_re : xbsIndex_r4/Reinterpret  force_arith_type=on  arith_type="Signed  (2's comp)"  force_bin_pt=on  bin_pt=7  block_type=reinterpret
      settings: infoedit="Changes signal type without altering the binary representation.   You can changed the signal between signed and unsigned, and relocate the binary point.<br><br>Hardware notes: In hardware this block costs nothing.<br><br>Example:  Suppose the input is 6 bits wide, signed, with 2 fractional bits, and the output is forced to unsigned with 0 fractional bits.  Then an input of -2.0 (1110.00 in binary 2's complement) becomes an output of 56 (111000 in binary)."
  slice_im : xbsIndex_r4/Slice  nbits=8  boolean_output=off  mode=Lower Bit Location + Width  bit1=0  base1=MSB of Input  bit0=0  base0=LSB of Input  dbl_ovrd=off  block_type=slice
  slice_re : xbsIndex_r4/Slice  nbits=8  boolean_output=off  mode=Upper Bit Location + Width  bit1=0  base1=MSB of Input  bit0=0  base0=LSB of Input  dbl_ovrd=off  block_type=slice
  re : Outport
  im : Outport  Port=2
  wires:
  c/1 -> slice_re/1, slice_im/1
  slice_im/1 -> force_im/1
  force_im/1 -> im/1
  force_re/1 -> re/1
  slice_re/1 -> force_re/1

== system xblock_half_band_Model/Subsystem/parallel_fir1/c_to_ri1 ==
  c : Inport
  force_im : xbsIndex_r4/Reinterpret  force_arith_type=on  arith_type="Signed  (2's comp)"  force_bin_pt=on  bin_pt=7  block_type=reinterpret
      settings: infoedit="Changes signal type without altering the binary representation.   You can changed the signal between signed and unsigned, and relocate the binary point.<br><br>Hardware notes: In hardware this block costs nothing.<br><br>Example:  Suppose the input is 6 bits wide, signed, with 2 fractional bits, and the output is forced to unsigned with 0 fractional bits.  Then an input of -2.0 (1110.00 in binary 2's complement) becomes an output of 56 (111000 in binary)."
  force_re : xbsIndex_r4/Reinterpret  force_arith_type=on  arith_type="Signed  (2's comp)"  force_bin_pt=on  bin_pt=7  block_type=reinterpret
      settings: infoedit="Changes signal type without altering the binary representation.   You can changed the signal between signed and unsigned, and relocate the binary point.<br><br>Hardware notes: In hardware this block costs nothing.<br><br>Example:  Suppose the input is 6 bits wide, signed, with 2 fractional bits, and the output is forced to unsigned with 0 fractional bits.  Then an input of -2.0 (1110.00 in binary 2's complement) becomes an output of 56 (111000 in binary)."
  slice_im : xbsIndex_r4/Slice  nbits=8  boolean_output=off  mode=Lower Bit Location + Width  bit1=0  base1=MSB of Input  bit0=0  base0=LSB of Input  dbl_ovrd=off  block_type=slice
  slice_re : xbsIndex_r4/Slice  nbits=8  boolean_output=off  mode=Upper Bit Location + Width  bit1=0  base1=MSB of Input  bit0=0  base0=LSB of Input  dbl_ovrd=off  block_type=slice
  re : Outport
  im : Outport  Port=2
  wires:
  c/1 -> slice_re/1, slice_im/1
  slice_im/1 -> force_im/1
  force_im/1 -> im/1
  force_re/1 -> re/1
  slice_re/1 -> force_re/1

== system xblock_half_band_Model/Subsystem/parallel_fir1/c_to_ri2 ==
  c : Inport
  force_im : xbsIndex_r4/Reinterpret  force_arith_type=on  arith_type="Signed  (2's comp)"  force_bin_pt=on  bin_pt=7  block_type=reinterpret
      settings: infoedit="Changes signal type without altering the binary representation.   You can changed the signal between signed and unsigned, and relocate the binary point.<br><br>Hardware notes: In hardware this block costs nothing.<br><br>Example:  Suppose the input is 6 bits wide, signed, with 2 fractional bits, and the output is forced to unsigned with 0 fractional bits.  Then an input of -2.0 (1110.00 in binary 2's complement) becomes an output of 56 (111000 in binary)."
  force_re : xbsIndex_r4/Reinterpret  force_arith_type=on  arith_type="Signed  (2's comp)"  force_bin_pt=on  bin_pt=7  block_type=reinterpret
      settings: infoedit="Changes signal type without altering the binary representation.   You can changed the signal between signed and unsigned, and relocate the binary point.<br><br>Hardware notes: In hardware this block costs nothing.<br><br>Example:  Suppose the input is 6 bits wide, signed, with 2 fractional bits, and the output is forced to unsigned with 0 fractional bits.  Then an input of -2.0 (1110.00 in binary 2's complement) becomes an output of 56 (111000 in binary)."
  slice_im : xbsIndex_r4/Slice  nbits=8  boolean_output=off  mode=Lower Bit Location + Width  bit1=0  base1=MSB of Input  bit0=0  base0=LSB of Input  dbl_ovrd=off  block_type=slice
  slice_re : xbsIndex_r4/Slice  nbits=8  boolean_output=off  mode=Upper Bit Location + Width  bit1=0  base1=MSB of Input  bit0=0  base0=LSB of Input  dbl_ovrd=off  block_type=slice
  re : Outport
  im : Outport  Port=2
  wires:
  c/1 -> slice_re/1, slice_im/1
  slice_im/1 -> force_im/1
  force_im/1 -> im/1
  force_re/1 -> re/1
  slice_re/1 -> force_re/1

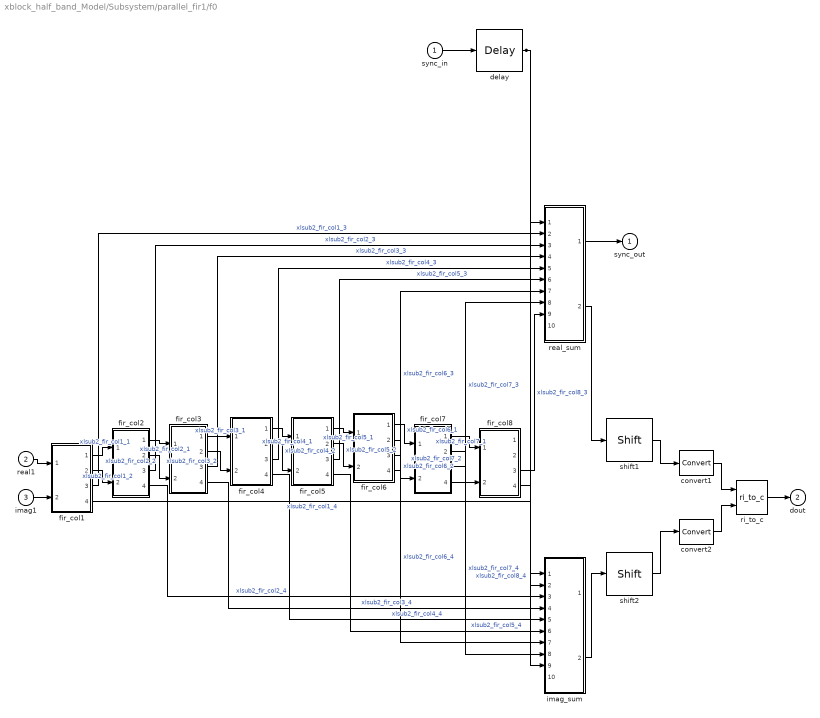
== system xblock_half_band_Model/Subsystem/parallel_fir1/f0 ==
  sync_in : Inport
  real1 : Inport  Port=2
  imag1 : Inport  Port=3
  convert1 : xbsIndex_r4/Convert  arith_type="Signed  (2's comp)"  n_bits=4  bin_pt=3  quantization=Truncate  overflow=Wrap  latency=1  dbl_ovrd=off  pipeline=off  block_type=convert
      settings: block_version=11.4
  convert2 : xbsIndex_r4/Convert  arith_type="Signed  (2's comp)"  n_bits=4  bin_pt=3  quantization=Truncate  overflow=Wrap  latency=1  dbl_ovrd=off  pipeline=off  block_type=convert
      settings: block_version=11.4
  delay : xbsIndex_r4/Delay  en=off  latency=3  dbl_ovrd=off  reg_retiming=off  block_type=delay
      settings: block_version=11.4
  fir_col1 : Subsystem
  fir_col2 : Subsystem
  fir_col3 : Subsystem
  fir_col4 : Subsystem
  fir_col5 : Subsystem
  fir_col6 : Subsystem
  fir_col7 : Subsystem
  fir_col8 : Subsystem
  imag_sum : Subsystem
  real_sum : Subsystem
  ri_to_c : casper_library_misc/ri_to_c  SystemSampleTime=-1
  shift1 : xbsIndex_r4/Shift  shift_dir=Left  shift_bits=1  en=off  latency=0  precision=Full  arith_type="Signed  (2's comp)"  n_bits=16  bin_pt=14  quantization=Truncate  overflow=Wrap  dbl_ovrd=off  block_type=shift
  shift2 : xbsIndex_r4/Shift  shift_dir=Left  shift_bits=1  en=off  latency=0  precision=Full  arith_type="Signed  (2's comp)"  n_bits=16  bin_pt=14  quantization=Truncate  overflow=Wrap  dbl_ovrd=off  block_type=shift
  sync_out : Outport
  dout : Outport  Port=2
  wires:
  delay/1 -> real_sum/1(sync), imag_sum/1(sync)
  imag_sum/2(dout) -> shift2/1
  shift1/1 -> convert1/1
  convert2/1 -> ri_to_c/2
  fir_col8/3(real_sum) -> real_sum/9(din_8)  "xlsub2_fir_col8_3"
  fir_col6/3(real_sum) -> real_sum/7(din_6)  "xlsub2_fir_col6_3"
  fir_col4/3(real_sum) -> real_sum/5(din_4)  "xlsub2_fir_col4_3"
  fir_col2/3(real_sum) -> real_sum/3(din_2)  "xlsub2_fir_col2_3"
  fir_col8/4(imag_sum) -> imag_sum/9(din_8)  "xlsub2_fir_col8_4"
  fir_col6/4(imag_sum) -> imag_sum/7(din_6)  "xlsub2_fir_col6_4"
  fir_col4/4(imag_sum) -> imag_sum/5(din_4)  "xlsub2_fir_col4_4"
  fir_col2/4(imag_sum) -> imag_sum/3(din_2)  "xlsub2_fir_col2_4"
  fir_col7/2(imag_out1) -> fir_col8/2(imag1)  "xlsub2_fir_col7_2"
  fir_col6/1(real_out1) -> fir_col7/1(real1)  "xlsub2_fir_col6_1"
  fir_col5/2(imag_out1) -> fir_col6/2(imag1)  "xlsub2_fir_col5_2"
  fir_col4/1(real_out1) -> fir_col5/1(real1)  "xlsub2_fir_col4_1"
  fir_col3/2(imag_out1) -> fir_col4/2(imag1)  "xlsub2_fir_col3_2"
  fir_col2/1(real_out1) -> fir_col3/1(real1)  "xlsub2_fir_col2_1"
  fir_col1/2(imag_out1) -> fir_col2/2(imag1)  "xlsub2_fir_col1_2"
  real1/1 -> fir_col1/1(real1)
  sync_in/1 -> delay/1
  imag1/1 -> fir_col1/2(imag1)
  fir_col1/1(real_out1) -> fir_col2/1(real1)  "xlsub2_fir_col1_1"
  fir_col2/2(imag_out1) -> fir_col3/2(imag1)  "xlsub2_fir_col2_2"
  fir_col3/1(real_out1) -> fir_col4/1(real1)  "xlsub2_fir_col3_1"
  fir_col4/2(imag_out1) -> fir_col5/2(imag1)  "xlsub2_fir_col4_2"
  fir_col5/1(real_out1) -> fir_col6/1(real1)  "xlsub2_fir_col5_1"
  fir_col6/2(imag_out1) -> fir_col7/2(imag1)  "xlsub2_fir_col6_2"
  fir_col7/1(real_out1) -> fir_col8/1(real1)  "xlsub2_fir_col7_1"
  fir_col1/4(imag_sum) -> imag_sum/2(din_1)  "xlsub2_fir_col1_4"
  fir_col3/4(imag_sum) -> imag_sum/4(din_3)  "xlsub2_fir_col3_4"
  fir_col5/4(imag_sum) -> imag_sum/6(din_5)  "xlsub2_fir_col5_4"
  fir_col7/4(imag_sum) -> imag_sum/8(din_7)  "xlsub2_fir_col7_4"
  fir_col1/3(real_sum) -> real_sum/2(din_1)  "xlsub2_fir_col1_3"
  fir_col3/3(real_sum) -> real_sum/4(din_3)  "xlsub2_fir_col3_3"
  fir_col5/3(real_sum) -> real_sum/6(din_5)  "xlsub2_fir_col5_3"
  fir_col7/3(real_sum) -> real_sum/8(din_7)  "xlsub2_fir_col7_3"
  real_sum/1(sync_out) -> sync_out/1
  convert1/1 -> ri_to_c/1
  ri_to_c/1 -> dout/1
  real_sum/2(dout) -> shift1/1
  shift2/1 -> convert2/1

== system xblock_half_band_Model/Subsystem/parallel_fir1/f0pf1 ==
  sync_in : Inport
  real1 : Inport  Port=2
  imag1 : Inport  Port=3
  convert1 : xbsIndex_r4/Convert  arith_type="Signed  (2's comp)"  n_bits=4  bin_pt=3  quantization=Truncate  overflow=Wrap  latency=1  dbl_ovrd=off  pipeline=off  block_type=convert
      settings: block_version=11.4
  convert2 : xbsIndex_r4/Convert  arith_type="Signed  (2's comp)"  n_bits=4  bin_pt=3  quantization=Truncate  overflow=Wrap  latency=1  dbl_ovrd=off  pipeline=off  block_type=convert
      settings: block_version=11.4
  delay : xbsIndex_r4/Delay  en=off  latency=3  dbl_ovrd=off  reg_retiming=off  block_type=delay
      settings: block_version=11.4
  fir_col1 : Subsystem
  fir_col2 : Subsystem
  fir_col3 : Subsystem
  fir_col4 : Subsystem
  fir_col5 : Subsystem
  imag_sum : Subsystem
  real_sum : Subsystem
  ri_to_c : casper_library_misc/ri_to_c  SystemSampleTime=-1
  shift1 : xbsIndex_r4/Shift  shift_dir=Left  shift_bits=1  en=off  latency=0  precision=Full  arith_type="Signed  (2's comp)"  n_bits=16  bin_pt=14  quantization=Truncate  overflow=Wrap  dbl_ovrd=off  block_type=shift
  shift2 : xbsIndex_r4/Shift  shift_dir=Left  shift_bits=1  en=off  latency=0  precision=Full  arith_type="Signed  (2's comp)"  n_bits=16  bin_pt=14  quantization=Truncate  overflow=Wrap  dbl_ovrd=off  block_type=shift
  sync_out : Outport
  dout : Outport  Port=2
  wires:
  delay/1 -> imag_sum/1(sync), real_sum/1(sync)
  imag_sum/2(dout) -> shift2/1
  shift1/1 -> convert1/1
  convert2/1 -> ri_to_c/2
  fir_col5/3(real_sum) -> real_sum/6(din_5)  "xlsub2_fir_col5_3"
  fir_col3/3(real_sum) -> real_sum/4(din_3)  "xlsub2_fir_col3_3"
  fir_col1/3(real_sum) -> real_sum/2(din_1)  "xlsub2_fir_col1_3"
  fir_col4/4(imag_sum) -> imag_sum/5(din_4)  "xlsub2_fir_col4_4"
  fir_col2/4(imag_sum) -> imag_sum/3(din_2)  "xlsub2_fir_col2_4"
  fir_col4/2(imag_out1) -> fir_col5/2(imag1)  "xlsub2_fir_col4_2"
  fir_col3/1(real_out1) -> fir_col4/1(real1)  "xlsub2_fir_col3_1"
  fir_col2/2(imag_out1) -> fir_col3/2(imag1)  "xlsub2_fir_col2_2"
  fir_col1/1(real_out1) -> fir_col2/1(real1)  "xlsub2_fir_col1_1"
  imag1/1 -> fir_col1/2(imag1)
  sync_in/1 -> delay/1
  real1/1 -> fir_col1/1(real1)
  fir_col1/2(imag_out1) -> fir_col2/2(imag1)  "xlsub2_fir_col1_2"
  fir_col2/1(real_out1) -> fir_col3/1(real1)  "xlsub2_fir_col2_1"
  fir_col3/2(imag_out1) -> fir_col4/2(imag1)  "xlsub2_fir_col3_2"
  fir_col4/1(real_out1) -> fir_col5/1(real1)  "xlsub2_fir_col4_1"
  fir_col1/4(imag_sum) -> imag_sum/2(din_1)  "xlsub2_fir_col1_4"
  fir_col3/4(imag_sum) -> imag_sum/4(din_3)  "xlsub2_fir_col3_4"
  fir_col5/4(imag_sum) -> imag_sum/6(din_5)  "xlsub2_fir_col5_4"
  fir_col2/3(real_sum) -> real_sum/3(din_2)  "xlsub2_fir_col2_3"
  fir_col4/3(real_sum) -> real_sum/5(din_4)  "xlsub2_fir_col4_3"
  real_sum/1(sync_out) -> sync_out/1
  convert1/1 -> ri_to_c/1
  ri_to_c/1 -> dout/1
  real_sum/2(dout) -> shift1/1
  shift2/1 -> convert2/1
